simulink model "Task_D_robs"  (R2022b)
settings: Solver=ode45  StartTime=0.0  StopTime=10.0  RelTol=1e-3
undefined symbols (not defined in the file): A_11, A_12, A_21, A_22, absolute_encoder_counts_per_revolution, B_1, B_2, init, J_r, K_ctr, K_I
libraries: simulink_extras x5, simulink x1
settings Model: Creator=tumisangramotlhwa  LastModifiedBy=tumisangramotlhwa

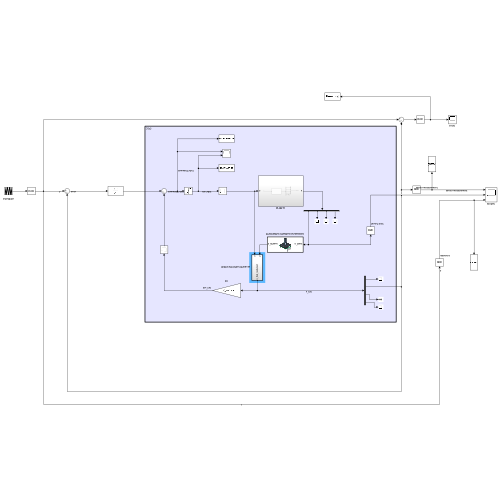
[thumbnail: Simulink's stored preview of the top-level diagram]
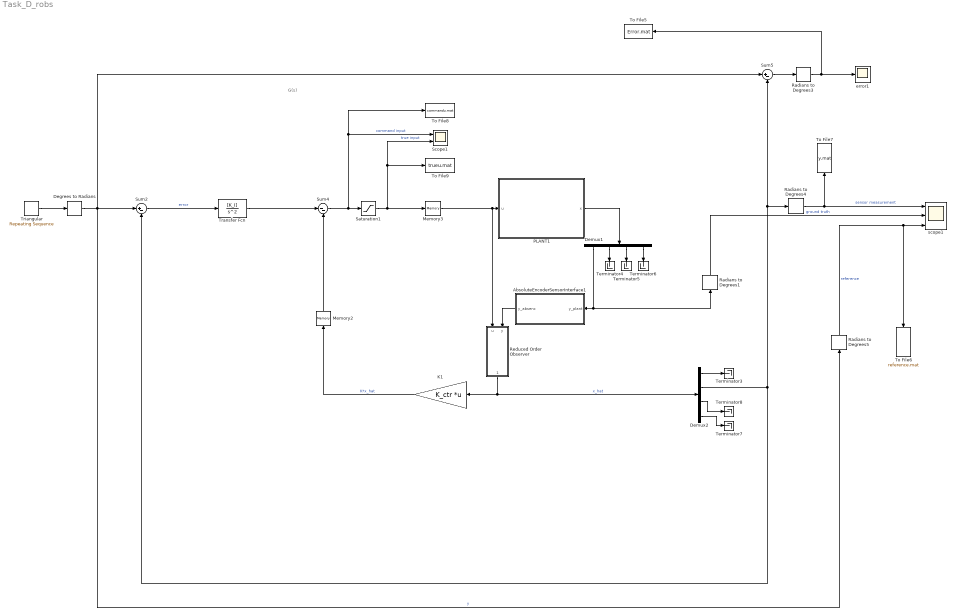
== system Task_D_robs ==
  note: G(s)
  " Triangular" : simulink/Sources/Repeating Sequence  rep_seq_t=[0 2 4]  rep_seq_y=[45 15 45]
  AbsoluteEncoderSensorInterface1 : Subsystem  TreatAsAtomicUnit=on
      mask Display: image('$imagefile'); % Use "Edit Image" on toolstrip to change.
  Degrees to Radians : simulink_extras/Transformations/Degrees to Radians
  Demux1 : Demux
  Demux2 : Demux
  K1 : Gain  Gain=K_ctr  Multiplication=Matrix(K*u) (u vector)
  Memory2 : Memory
  Memory3 : Memory
  PLANT1 : Subsystem
  Radians to Degrees{1,3..5} (4 alike) : simulink_extras/Transformations/Radians to Degrees
  Reduced Order Observer : Subsystem  TreatAsAtomicUnit=on
  Saturation1 : Saturate  UpperLimit=6  LowerLimit=-6
  Scope1 : Scope  NumInputPorts=2
  Sum2 : Sum  Inputs=|+-
  Sum4 : Sum  Inputs=|--
  Sum5 : Sum  Inputs=|+-
  Terminator{3..8} (6 alike) : Terminator
  To File5 : ToFile  Filename=Error.mat  MatrixName=Error  SaveFormat=Timeseries
  To File6 : ToFile  Filename=reference.mat  MatrixName=reference  SaveFormat=Timeseries
  To File7 : ToFile  Filename=y.mat  MatrixName=y  SaveFormat=Timeseries
  To File8 : ToFile  Filename=commandu.mat  MatrixName=commandu  SaveFormat=Timeseries
  To File9 : ToFile  Filename=trueu.mat  MatrixName=trueu  SaveFormat=Timeseries
  Transfer Fcn : TransferFcn  Numerator=[K_I]  Denominator=[1 0 0]
  error1 : Scope
  scope1 : Scope  NumInputPorts=3
  wires:
  Demux1/1 -> Radians to Degrees1/1, AbsoluteEncoderSensorInterface1/1(y_plant)
  Radians to Degrees3/1 -> error1/1, To File5/1
  Reduced Order Observer/1(x_hat_reduced) -> Demux2/1, K1/1  "x_hat"
  Radians to Degrees4/1 -> scope1/1, To File7/1  "sensor measurement"
  Demux2/3 -> Terminator8/1
  Saturation1/1 -> Memory3/1, To File9/1, Scope1/2  "true input"
  Memory3/1 -> Reduced Order Observer/1(u), PLANT1/1(u)
  Demux1/4 -> Terminator6/1
  Demux2/4 -> Terminator7/1
  Sum5/1 -> Radians to Degrees3/1
  Radians to Degrees5/1 -> scope1/3, To File6/1  "reference"
  Memory2/1 -> Sum4/2
  Sum4/1 -> Saturation1/1, To File8/1, Scope1/1  "command input"
  Demux1/3 -> Terminator5/1
  PLANT1/1(x) -> Demux1/1
  Demux1/2 -> Terminator4/1
  Degrees to Radians/1 -> Radians to Degrees5/1, Sum5/1, Sum2/1  "y"
  AbsoluteEncoderSensorInterface1/1(y_absenc) -> Reduced Order Observer/2(y)
  Demux2/2 -> Sum5/2, Radians to Degrees4/1, Sum2/2
  Sum2/1 -> Transfer Fcn/1  "error"
  K1/1 -> Memory2/1  "K*x_hat"
  Demux2/1 -> Terminator3/1
  Radians to Degrees1/1 -> scope1/2  "ground truth"
  Transfer Fcn/1 -> Sum4/1
  " Triangular"/1 -> Degrees to Radians/1

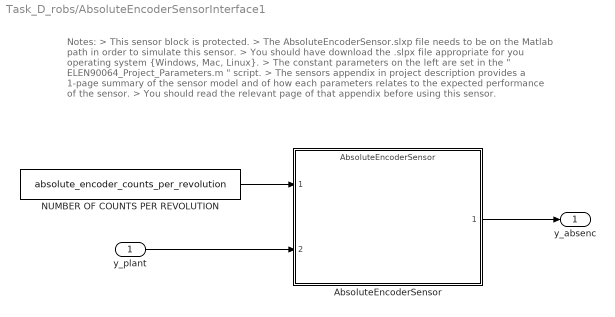
== system Task_D_robs/AbsoluteEncoderSensorInterface1 ==
  note: Notes:
      | > This sensor block is protected.
      | > The AbsoluteEncoderSensor.slxp file needs to be on the Matlab path in order to simulate this sensor.
      | > You should have download the .slpx file appropriate for you operating system {Windows, Mac, Linux}.
      | > The constant parameters on the left are set in the " ELEN90064_Project_Parameters.m " script.
      | > The sensors appendix in project description provides a 1-page summary of the sensor model and of how each parameters relates to the expected performance of the sensor.
      | > You should read the relevant page of that appendix before using this sensor.
  y_plant : Inport
  AbsoluteEncoderSensor : ModelReference  ModelNameDialog=AbsoluteEncoderSensor.slxp  ModelReferenceVersion=1.16  CopyOfModelProtected=on
  NUMBER OF COUNTS PER REVOLUTION : Constant  Value=absolute_encoder_counts_per_revolution
  y_absenc : Outport
  wires:
  NUMBER OF COUNTS PER REVOLUTION/1 -> AbsoluteEncoderSensor/1
  y_plant/1 -> AbsoluteEncoderSensor/2
  AbsoluteEncoderSensor/1 -> y_absenc/1

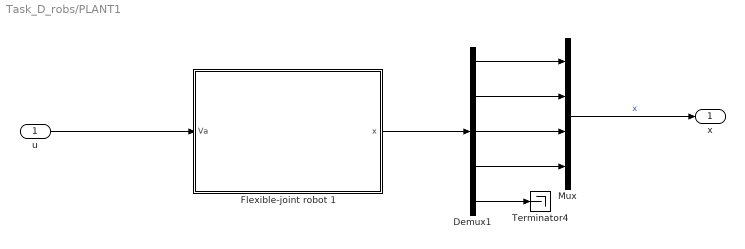
== system Task_D_robs/PLANT1 ==
  u : Inport
  Demux1 : Demux  Outputs=5
  Flexible-joint robot 1 : Subsystem
      mask Display: image('$imagefile'); % Use "Edit Image" on toolstrip to change.
  Mux : Mux
  Terminator4 : Terminator
  x : Outport
  wires:
  Mux/1 -> x/1  "x"
  Demux1/4 -> Mux/4
  Flexible-joint robot 1/1(x) -> Demux1/1
  Demux1/3 -> Mux/3
  Demux1/2 -> Mux/2
  Demux1/1 -> Mux/1
  Demux1/5 -> Terminator4/1
  u/1 -> Flexible-joint robot 1/1(Va)

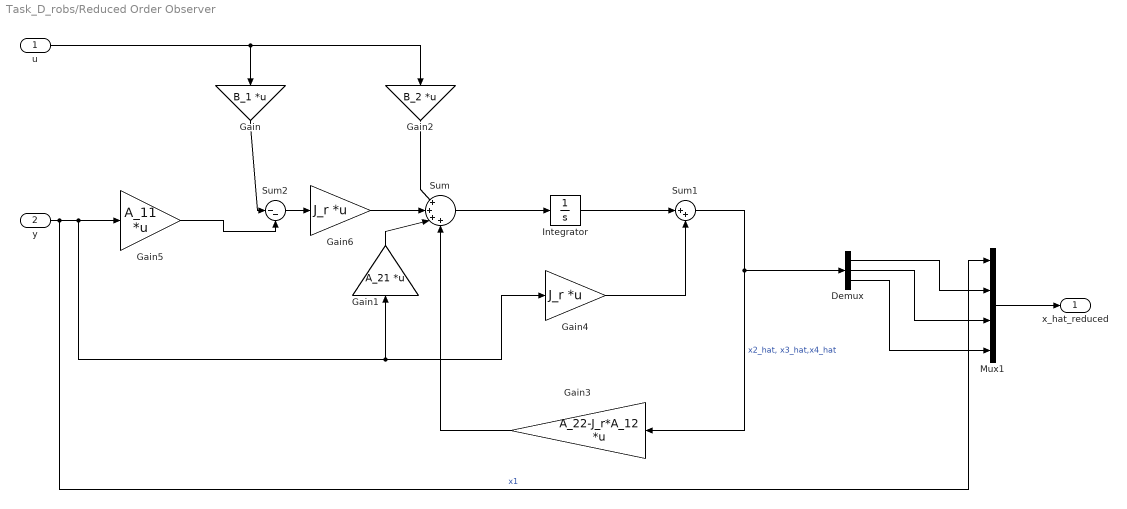
== system Task_D_robs/Reduced Order Observer ==
  u : Inport
  y : Inport  Port=2
  Demux : Demux  Outputs=3
  Gain : Gain  Gain=B_1  Multiplication=Matrix(K*u) (u vector)
  Gain1 : Gain  Gain=A_21  Multiplication=Matrix(K*u) (u vector)
  Gain2 : Gain  Gain=B_2  Multiplication=Matrix(K*u) (u vector)
  Gain3 : Gain  Gain=A_22-J_r*A_12  Multiplication=Matrix(K*u) (u vector)
  Gain4 : Gain  Gain=J_r  Multiplication=Matrix(K*u) (u vector)
  Gain5 : Gain  Gain=A_11  Multiplication=Matrix(K*u) (u vector)
  Gain6 : Gain  Gain=J_r  Multiplication=Matrix(K*u) (u vector)
  Integrator : Integrator
  Mux1 : Mux
  Sum : Sum  Inputs=|++++
  Sum1 : Sum  Inputs=|++
  Sum2 : Sum  Inputs=|--
  x_hat_reduced : Outport
  wires:
  u/1 -> Gain2/1, Gain/1
  y/1 -> Mux1/1, Gain5/1, Gain4/1, Gain1/1  "x1"
  Sum/1 -> Integrator/1
  Gain6/1 -> Sum/2
  Gain1/1 -> Sum/3
  Gain/1 -> Sum2/1
  Gain5/1 -> Sum2/2
  Gain2/1 -> Sum/1
  Integrator/1 -> Sum1/1
  Gain4/1 -> Sum1/2
  Gain3/1 -> Sum/4
  Sum1/1 -> Demux/1, Gain3/1  "x2_hat, x3_hat,x4_hat"
  Sum2/1 -> Gain6/1
  Mux1/1 -> x_hat_reduced/1
  Demux/1 -> Mux1/2
  Demux/2 -> Mux1/3
  Demux/3 -> Mux1/4

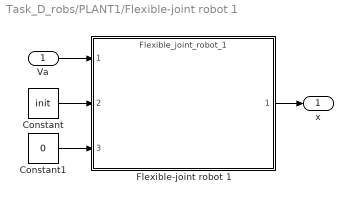
== system Task_D_robs/PLANT1/Flexible-joint robot 1 ==
  Va : Inport
  Constant : Constant  Value=init
  Constant1 : Constant  Value=0
  Flexible-joint robot 1 : ModelReference  ModelNameDialog=Flexible_joint_robot_1  ModelReferenceVersion=1.63  CopyOfModelProtected=on
  x : Outport
  wires:
  Constant/1 -> Flexible-joint robot 1/2
  Constant1/1 -> Flexible-joint robot 1/3
  Flexible-joint robot 1/1 -> x/1
  Va/1 -> Flexible-joint robot 1/1
